simulink model "Thermal_Plant_model"  (R2025b)
settings: Solver=FixedStepDiscrete  StartTime=0.0  StopTime=200  FixedStep=0.1  RelTol=1e-3
libraries: slpidlib x4
settings Model: Creator=MFM  LastModifiedBy=MFM

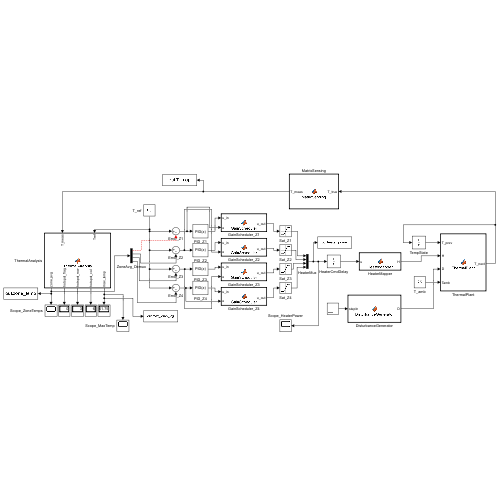
[thumbnail: Simulink's stored preview of the top-level diagram]
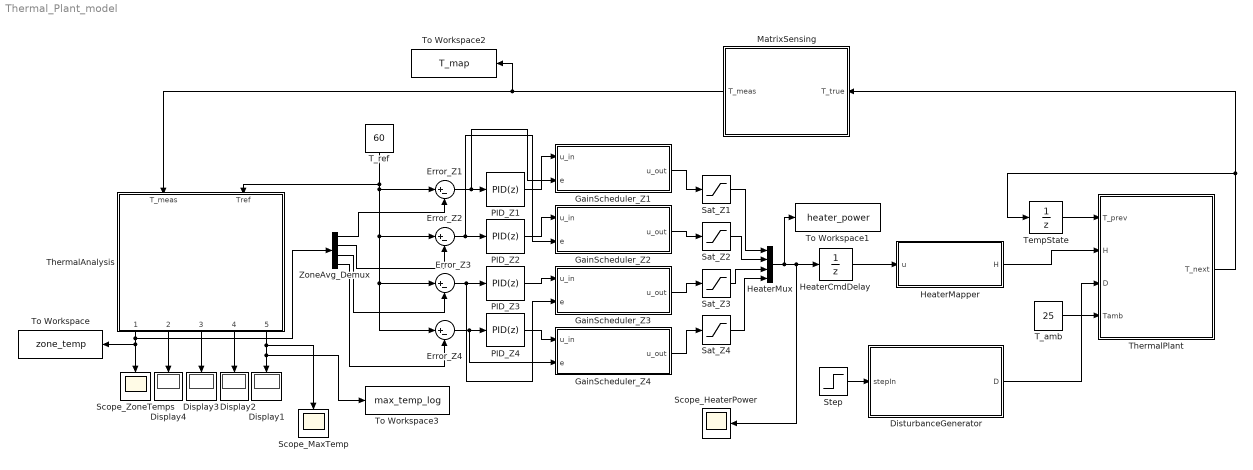
== system Thermal_Plant_model ==
  Display{1..4} (4 alike) : Display
  DisturbanceGenerator : MATLAB Function  TreatAsAtomicUnit=on
  Error_Z{1..4} (4 alike) : Sum  Inputs=|+-
  GainScheduler_Z1 : MATLAB Function  TreatAsAtomicUnit=on
  GainScheduler_Z2 : MATLAB Function  TreatAsAtomicUnit=on
  GainScheduler_Z3 : MATLAB Function  TreatAsAtomicUnit=on
  GainScheduler_Z4 : MATLAB Function  TreatAsAtomicUnit=on
  HeaterCmdDelay : UnitDelay  InitialCondition=[0 0 0 0]  SampleTime=-1  HasFrameUpgradeWarning=on
  HeaterMapper : MATLAB Function  TreatAsAtomicUnit=on
  HeaterMux : Mux
  MatrixSensing : MATLAB Function  TreatAsAtomicUnit=on
  PID_Z1 : slpidlib/PID Controller  Controller=PID  Form=Parallel  TimeDomain=Discrete-time  UseExternalTs=off  SampleTime=0.1  IntegratorMethod=Forward Euler  FilterMethod=Forward Euler  ControllerParametersSource=internal  P=2.5  I=1.2  UseKiTs=off  D=0.000  UseExternalDerivativeSource=off  N=100  UseFilter=on  TunerSelectOption=Transfer Function Based (PID Tuner App)  InitialConditionSource=internal  InitialConditionForIntegrator=0  InitialConditionForFilter=0  DifferentiatorICPrevScaledInput=0  ExternalReset=none  TrackingMode=off  Kt=1  LimitOutput=off  SatLimitsSource=internal  UpperSaturationLimit=inf  LowerSaturationLimit=-inf  LinearizeAsGain=on  AntiWindupMode=none  Kb=1  LimitIntegrator=off  UpperIntegratorSaturationLimit=inf  LowerIntegratorSaturationLimit=-inf  POutMin=[]  POutMax=[]  IOutMin=[]  IOutMax=[]  DOutMin=[]  DOutMax=[]  NOutMin=[]  NOutMax=[]  SumOutMin=[]  SumOutMax=[]  SaturationOutMin=[]  SaturationOutMax=[]  PParamMin=[]  PParamMax=[]  IParamMin=[]  IParamMax=[]  DParamMin=[]  DParamMax=[]  NParamMin=[]  NParamMax=[]  KbParamMin=[]  KbParamMax=[]  KtParamMin=[]  KtParamMax=[]  KbOutMin=[]  KbOutMax=[]  KtOutMin=[]  KtOutMax=[]  IntegratorOutMin=[]  IntegratorOutMax=[]  FilterOutMin=[]  FilterOutMax=[]  SumI1OutMin=[]  SumI1OutMax=[]  SumI2OutMin=[]  SumI2OutMax=[]  SumI3OutMin=[]  SumI3OutMax=[]  SumI4OutMin=[]  SumI4OutMax=[]  SumDOutMin=[]  SumDOutMax=[]  DifferentiatorOutMin=[]  DifferentiatorOutMax=[]  FilterDiffOutCoefMin=[]  FilterDiffOutCoefMax=[]  ReciprocalOutMin=[]  ReciprocalOutMax=[]  SumDenOutMin=[]  SumDenOutMax=[]  SumNumOutMin=[]  SumNumOutMax=[]  DivideOutMin=[]  DivideOutMax=[]  UdiffTsProdOutMin=[]  UdiffTsProdOutMax=[]  NTsProdOutMin=[]  NTsProdOutMax=[]  UintegralTsProdOutMin=[]  UintegralTsProdOutMax=[]  UngainTsProdOutMin=[]  UngainTsProdOutMax=[]  ClampingZeroOutDataTypeStr=Inherit: Inherit via back propagation  ClampingZeroOutMin=[]  ClampingZeroOutMax=[]  FilterDenConstantOutDataTypeStr=Inherit: Inherit via back propagation  FilterDenConstantOutMin=[]  FilterDenConstantOutMax=[]  PCopyOutDataTypeStr=Inherit: Inherit via back propagation  PCopyOutMin=[]  PCopyOutMax=[]  NCopyOutDataTypeStr=Inherit: Inherit via back propagation  NCopyOutMin=[]  NCopyOutMax=[]  IntegratorContinuousStateAttributes=''  IntegratorStateMustResolveToSignalObject=off  IntegratorRTWStateStorageClass=Auto  FilterContinuousStateAttributes=''  FilterStateMustResolveToSignalObject=off  FilterRTWStateStorageClass=Auto  ParallelPVariant=InternalParameters  IdealPVariant=Disabled  IVariant=InternalParameters  DVariant=InternalParameters  IntegratorVariant=Discrete  SatVariant=Disabled  AWVariant=Passthrough  PCopyVariant=Disabled  TRVariant=Disabled  FdbkBlocksVariant=Forward  IdealPFdbkVariant=Disabled  SatFdbkVariant=Disabled  DerivativeFilterVariant=ForwardEulerFilter  NVariant=InternalParameters  NCopyVariant=Disabled  FilterICVariant=InternalICsFilter  IntegratorICVariant=InternalICs  ExternalResetVariant=Disabled  TRSumVariant=Passthrough  SumFdbkVariant=Disabled  SumVariant=Sum_PID  TsampFilterVariant=InternalTs  TsampNgainVariant=Passthrough  TsampIntegralVariant=Disabled_SignalSpec  ExternalSaturationOutDataTypeStr=Inherit: Same as second input  DerivativeSourceVariant=ErrorSignal  PreIntVariant=InternalPreInt
  PID_Z2 : slpidlib/PID Controller  Controller=PID  Form=Parallel  TimeDomain=Discrete-time  UseExternalTs=off  SampleTime=0.1  IntegratorMethod=Forward Euler  FilterMethod=Forward Euler  ControllerParametersSource=internal  P=2.5  I=1.2  UseKiTs=off  D=0.0  UseExternalDerivativeSource=off  N=100  UseFilter=on  TunerSelectOption=Transfer Function Based (PID Tuner App)  InitialConditionSource=internal  InitialConditionForIntegrator=0  InitialConditionForFilter=0  DifferentiatorICPrevScaledInput=0  ExternalReset=none  TrackingMode=off  Kt=1  LimitOutput=off  SatLimitsSource=internal  UpperSaturationLimit=inf  LowerSaturationLimit=-inf  LinearizeAsGain=on  AntiWindupMode=none  Kb=1  LimitIntegrator=off  UpperIntegratorSaturationLimit=inf  LowerIntegratorSaturationLimit=-inf  POutMin=[]  POutMax=[]  IOutMin=[]  IOutMax=[]  DOutMin=[]  DOutMax=[]  NOutMin=[]  NOutMax=[]  SumOutMin=[]  SumOutMax=[]  SaturationOutMin=[]  SaturationOutMax=[]  PParamMin=[]  PParamMax=[]  IParamMin=[]  IParamMax=[]  DParamMin=[]  DParamMax=[]  NParamMin=[]  NParamMax=[]  KbParamMin=[]  KbParamMax=[]  KtParamMin=[]  KtParamMax=[]  KbOutMin=[]  KbOutMax=[]  KtOutMin=[]  KtOutMax=[]  IntegratorOutMin=[]  IntegratorOutMax=[]  FilterOutMin=[]  FilterOutMax=[]  SumI1OutMin=[]  SumI1OutMax=[]  SumI2OutMin=[]  SumI2OutMax=[]  SumI3OutMin=[]  SumI3OutMax=[]  SumI4OutMin=[]  SumI4OutMax=[]  SumDOutMin=[]  SumDOutMax=[]  DifferentiatorOutMin=[]  DifferentiatorOutMax=[]  FilterDiffOutCoefMin=[]  FilterDiffOutCoefMax=[]  ReciprocalOutMin=[]  ReciprocalOutMax=[]  SumDenOutMin=[]  SumDenOutMax=[]  SumNumOutMin=[]  SumNumOutMax=[]  DivideOutMin=[]  DivideOutMax=[]  UdiffTsProdOutMin=[]  UdiffTsProdOutMax=[]  NTsProdOutMin=[]  NTsProdOutMax=[]  UintegralTsProdOutMin=[]  UintegralTsProdOutMax=[]  UngainTsProdOutMin=[]  UngainTsProdOutMax=[]  ClampingZeroOutDataTypeStr=Inherit: Inherit via back propagation  ClampingZeroOutMin=[]  ClampingZeroOutMax=[]  FilterDenConstantOutDataTypeStr=Inherit: Inherit via back propagation  FilterDenConstantOutMin=[]  FilterDenConstantOutMax=[]  PCopyOutDataTypeStr=Inherit: Inherit via back propagation  PCopyOutMin=[]  PCopyOutMax=[]  NCopyOutDataTypeStr=Inherit: Inherit via back propagation  NCopyOutMin=[]  NCopyOutMax=[]  IntegratorContinuousStateAttributes=''  IntegratorStateMustResolveToSignalObject=off  IntegratorRTWStateStorageClass=Auto  FilterContinuousStateAttributes=''  FilterStateMustResolveToSignalObject=off  FilterRTWStateStorageClass=Auto  ParallelPVariant=InternalParameters  IdealPVariant=Disabled  IVariant=InternalParameters  DVariant=InternalParameters  IntegratorVariant=Discrete  SatVariant=Disabled  AWVariant=Passthrough  PCopyVariant=Disabled  TRVariant=Disabled  FdbkBlocksVariant=Forward  IdealPFdbkVariant=Disabled  SatFdbkVariant=Disabled  DerivativeFilterVariant=ForwardEulerFilter  NVariant=InternalParameters  NCopyVariant=Disabled  FilterICVariant=InternalICsFilter  IntegratorICVariant=InternalICs  ExternalResetVariant=Disabled  TRSumVariant=Passthrough  SumFdbkVariant=Disabled  SumVariant=Sum_PID  TsampFilterVariant=InternalTs  TsampNgainVariant=Passthrough  TsampIntegralVariant=Disabled_SignalSpec  ExternalSaturationOutDataTypeStr=Inherit: Same as second input  DerivativeSourceVariant=ErrorSignal  PreIntVariant=InternalPreInt
  PID_Z3 : slpidlib/PID Controller  Controller=PID  Form=Parallel  TimeDomain=Discrete-time  UseExternalTs=off  SampleTime=0.1  IntegratorMethod=Forward Euler  FilterMethod=Forward Euler  ControllerParametersSource=internal  P=2.5  I=1.2  UseKiTs=off  D=0  UseExternalDerivativeSource=off  N=100  UseFilter=on  TunerSelectOption=Transfer Function Based (PID Tuner App)  InitialConditionSource=internal  InitialConditionForIntegrator=0  InitialConditionForFilter=0  DifferentiatorICPrevScaledInput=0  ExternalReset=none  TrackingMode=off  Kt=1  LimitOutput=off  SatLimitsSource=internal  UpperSaturationLimit=inf  LowerSaturationLimit=-inf  LinearizeAsGain=on  AntiWindupMode=none  Kb=1  LimitIntegrator=off  UpperIntegratorSaturationLimit=inf  LowerIntegratorSaturationLimit=-inf  POutMin=[]  POutMax=[]  IOutMin=[]  IOutMax=[]  DOutMin=[]  DOutMax=[]  NOutMin=[]  NOutMax=[]  SumOutMin=[]  SumOutMax=[]  SaturationOutMin=[]  SaturationOutMax=[]  PParamMin=[]  PParamMax=[]  IParamMin=[]  IParamMax=[]  DParamMin=[]  DParamMax=[]  NParamMin=[]  NParamMax=[]  KbParamMin=[]  KbParamMax=[]  KtParamMin=[]  KtParamMax=[]  KbOutMin=[]  KbOutMax=[]  KtOutMin=[]  KtOutMax=[]  IntegratorOutMin=[]  IntegratorOutMax=[]  FilterOutMin=[]  FilterOutMax=[]  SumI1OutMin=[]  SumI1OutMax=[]  SumI2OutMin=[]  SumI2OutMax=[]  SumI3OutMin=[]  SumI3OutMax=[]  SumI4OutMin=[]  SumI4OutMax=[]  SumDOutMin=[]  SumDOutMax=[]  DifferentiatorOutMin=[]  DifferentiatorOutMax=[]  FilterDiffOutCoefMin=[]  FilterDiffOutCoefMax=[]  ReciprocalOutMin=[]  ReciprocalOutMax=[]  SumDenOutMin=[]  SumDenOutMax=[]  SumNumOutMin=[]  SumNumOutMax=[]  DivideOutMin=[]  DivideOutMax=[]  UdiffTsProdOutMin=[]  UdiffTsProdOutMax=[]  NTsProdOutMin=[]  NTsProdOutMax=[]  UintegralTsProdOutMin=[]  UintegralTsProdOutMax=[]  UngainTsProdOutMin=[]  UngainTsProdOutMax=[]  ClampingZeroOutDataTypeStr=Inherit: Inherit via back propagation  ClampingZeroOutMin=[]  ClampingZeroOutMax=[]  FilterDenConstantOutDataTypeStr=Inherit: Inherit via back propagation  FilterDenConstantOutMin=[]  FilterDenConstantOutMax=[]  PCopyOutDataTypeStr=Inherit: Inherit via back propagation  PCopyOutMin=[]  PCopyOutMax=[]  NCopyOutDataTypeStr=Inherit: Inherit via back propagation  NCopyOutMin=[]  NCopyOutMax=[]  IntegratorContinuousStateAttributes=''  IntegratorStateMustResolveToSignalObject=off  IntegratorRTWStateStorageClass=Auto  FilterContinuousStateAttributes=''  FilterStateMustResolveToSignalObject=off  FilterRTWStateStorageClass=Auto  ParallelPVariant=InternalParameters  IdealPVariant=Disabled  IVariant=InternalParameters  DVariant=InternalParameters  IntegratorVariant=Discrete  SatVariant=Disabled  AWVariant=Passthrough  PCopyVariant=Disabled  TRVariant=Disabled  FdbkBlocksVariant=Forward  IdealPFdbkVariant=Disabled  SatFdbkVariant=Disabled  DerivativeFilterVariant=ForwardEulerFilter  NVariant=InternalParameters  NCopyVariant=Disabled  FilterICVariant=InternalICsFilter  IntegratorICVariant=InternalICs  ExternalResetVariant=Disabled  TRSumVariant=Passthrough  SumFdbkVariant=Disabled  SumVariant=Sum_PID  TsampFilterVariant=InternalTs  TsampNgainVariant=Passthrough  TsampIntegralVariant=Disabled_SignalSpec  ExternalSaturationOutDataTypeStr=Inherit: Same as second input  DerivativeSourceVariant=ErrorSignal  PreIntVariant=InternalPreInt
  PID_Z4 : slpidlib/PID Controller  Controller=PID  Form=Parallel  TimeDomain=Discrete-time  UseExternalTs=off  SampleTime=0.1  IntegratorMethod=Forward Euler  FilterMethod=Forward Euler  ControllerParametersSource=internal  P=2.5  I=1.2  UseKiTs=off  D=0  UseExternalDerivativeSource=off  N=100  UseFilter=on  TunerSelectOption=Transfer Function Based (PID Tuner App)  InitialConditionSource=internal  InitialConditionForIntegrator=0  InitialConditionForFilter=0  DifferentiatorICPrevScaledInput=0  ExternalReset=none  TrackingMode=off  Kt=1  LimitOutput=off  SatLimitsSource=internal  UpperSaturationLimit=inf  LowerSaturationLimit=-inf  LinearizeAsGain=on  AntiWindupMode=none  Kb=1  LimitIntegrator=off  UpperIntegratorSaturationLimit=inf  LowerIntegratorSaturationLimit=-inf  POutMin=[]  POutMax=[]  IOutMin=[]  IOutMax=[]  DOutMin=[]  DOutMax=[]  NOutMin=[]  NOutMax=[]  SumOutMin=[]  SumOutMax=[]  SaturationOutMin=[]  SaturationOutMax=[]  PParamMin=[]  PParamMax=[]  IParamMin=[]  IParamMax=[]  DParamMin=[]  DParamMax=[]  NParamMin=[]  NParamMax=[]  KbParamMin=[]  KbParamMax=[]  KtParamMin=[]  KtParamMax=[]  KbOutMin=[]  KbOutMax=[]  KtOutMin=[]  KtOutMax=[]  IntegratorOutMin=[]  IntegratorOutMax=[]  FilterOutMin=[]  FilterOutMax=[]  SumI1OutMin=[]  SumI1OutMax=[]  SumI2OutMin=[]  SumI2OutMax=[]  SumI3OutMin=[]  SumI3OutMax=[]  SumI4OutMin=[]  SumI4OutMax=[]  SumDOutMin=[]  SumDOutMax=[]  DifferentiatorOutMin=[]  DifferentiatorOutMax=[]  FilterDiffOutCoefMin=[]  FilterDiffOutCoefMax=[]  ReciprocalOutMin=[]  ReciprocalOutMax=[]  SumDenOutMin=[]  SumDenOutMax=[]  SumNumOutMin=[]  SumNumOutMax=[]  DivideOutMin=[]  DivideOutMax=[]  UdiffTsProdOutMin=[]  UdiffTsProdOutMax=[]  NTsProdOutMin=[]  NTsProdOutMax=[]  UintegralTsProdOutMin=[]  UintegralTsProdOutMax=[]  UngainTsProdOutMin=[]  UngainTsProdOutMax=[]  ClampingZeroOutDataTypeStr=Inherit: Inherit via back propagation  ClampingZeroOutMin=[]  ClampingZeroOutMax=[]  FilterDenConstantOutDataTypeStr=Inherit: Inherit via back propagation  FilterDenConstantOutMin=[]  FilterDenConstantOutMax=[]  PCopyOutDataTypeStr=Inherit: Inherit via back propagation  PCopyOutMin=[]  PCopyOutMax=[]  NCopyOutDataTypeStr=Inherit: Inherit via back propagation  NCopyOutMin=[]  NCopyOutMax=[]  IntegratorContinuousStateAttributes=''  IntegratorStateMustResolveToSignalObject=off  IntegratorRTWStateStorageClass=Auto  FilterContinuousStateAttributes=''  FilterStateMustResolveToSignalObject=off  FilterRTWStateStorageClass=Auto  ParallelPVariant=InternalParameters  IdealPVariant=Disabled  IVariant=InternalParameters  DVariant=InternalParameters  IntegratorVariant=Discrete  SatVariant=Disabled  AWVariant=Passthrough  PCopyVariant=Disabled  TRVariant=Disabled  FdbkBlocksVariant=Forward  IdealPFdbkVariant=Disabled  SatFdbkVariant=Disabled  DerivativeFilterVariant=ForwardEulerFilter  NVariant=InternalParameters  NCopyVariant=Disabled  FilterICVariant=InternalICsFilter  IntegratorICVariant=InternalICs  ExternalResetVariant=Disabled  TRSumVariant=Passthrough  SumFdbkVariant=Disabled  SumVariant=Sum_PID  TsampFilterVariant=InternalTs  TsampNgainVariant=Passthrough  TsampIntegralVariant=Disabled_SignalSpec  ExternalSaturationOutDataTypeStr=Inherit: Same as second input  DerivativeSourceVariant=ErrorSignal  PreIntVariant=InternalPreInt
  Sat_Z{1..4} (4 alike) : Saturate  UpperLimit=100  LowerLimit=0
  Scope_HeaterPower : Scope
      settings: ActiveDisplayYMinimum=22.165592278395341  ActiveDisplayYMaximum=108.64826752462274
  Scope_MaxTemp : Scope
      settings: ActiveDisplayYMinimum=19.949054372354  ActiveDisplayYMaximum=70.261232158835853  DataLoggingVariableName=ScopeData2
  Scope_ZoneTemps : Scope
      settings: ActiveDisplayYMinimum=19.949054372354  ActiveDisplayYMaximum=70.261232158835853
  Step : Step  Time=10  SampleTime=0
  T_amb : Constant  Value=25
  T_ref : Constant  Value=60
  TempState : UnitDelay  InitialCondition=25*ones(6,8)  SampleTime=-1  HasFrameUpgradeWarning=on
  ThermalAnalysis : MATLAB Function  TreatAsAtomicUnit=on
  ThermalPlant : MATLAB Function  TreatAsAtomicUnit=on
  To Workspace : ToWorkspace  VariableName=zone_temp  SaveFormat=Structure With Time  SampleTime=-1
  To Workspace1 : ToWorkspace  VariableName=heater_power  SaveFormat=Structure With Time  SampleTime=-1
  To Workspace2 : ToWorkspace  VariableName=T_map  SaveFormat=Timeseries  SampleTime=-1
  To Workspace3 : ToWorkspace  VariableName=max_temp_log  SaveFormat=Structure With Time  SampleTime=-1
  ZoneAvg_Demux : Demux
  wires:
  T_ref/1 -> Error_Z3/1, Error_Z4/1, Error_Z2/1, Error_Z1/1, ThermalAnalysis/2(Tref)
  ZoneAvg_Demux/1 -> Error_Z1/2
  ZoneAvg_Demux/2 -> Error_Z2/2
  ZoneAvg_Demux/3 -> Error_Z3/2
  ZoneAvg_Demux/4 -> Error_Z4/2
  Sat_Z4/1 -> HeaterMux/4
  Sat_Z3/1 -> HeaterMux/3
  Sat_Z2/1 -> HeaterMux/2
  Sat_Z1/1 -> HeaterMux/1
  Step/1 -> DisturbanceGenerator/1(stepIn)
  T_amb/1 -> ThermalPlant/4(Tamb)
  TempState/1 -> ThermalPlant/1(T_prev)
  HeaterMapper/1(H) -> ThermalPlant/2(H)
  DisturbanceGenerator/1(D) -> ThermalPlant/3(D)
  ThermalPlant/1(T_next) -> TempState/1, MatrixSensing/1(T_true)
  MatrixSensing/1(T_meas) -> To Workspace2/1, ThermalAnalysis/1(T_meas)
  ThermalAnalysis/5(max_temp) -> Scope_MaxTemp/1, To Workspace3/1, Display1/1
  ThermalAnalysis/4(hotspot_col) -> Display2/1
  ThermalAnalysis/3(hotspot_row) -> Display3/1
  ThermalAnalysis/2(hotspot_flag) -> Display4/1
  Error_Z4/1 -> GainScheduler_Z4/2(e), PID_Z4/1
  Error_Z2/1 -> GainScheduler_Z2/2(e), PID_Z2/1
  Error_Z3/1 -> GainScheduler_Z3/2(e), PID_Z3/1
  Error_Z1/1 -> GainScheduler_Z1/2(e), PID_Z1/1
  HeaterMux/1 -> To Workspace1/1, Scope_HeaterPower/1, HeaterCmdDelay/1
  HeaterCmdDelay/1 -> HeaterMapper/1(u)
  ThermalAnalysis/1(zone_avg) -> Scope_ZoneTemps/1, To Workspace/1, ZoneAvg_Demux/1
  GainScheduler_Z1/1(u_out) -> Sat_Z1/1
  PID_Z1/1 -> GainScheduler_Z1/1(u_in)
  PID_Z2/1 -> GainScheduler_Z2/1(u_in)
  PID_Z3/1 -> GainScheduler_Z3/1(u_in)
  PID_Z4/1 -> GainScheduler_Z4/1(u_in)
  GainScheduler_Z2/1(u_out) -> Sat_Z2/1
  GainScheduler_Z3/1(u_out) -> Sat_Z3/1
  GainScheduler_Z4/1(u_out) -> Sat_Z4/1

== matlab function Thermal_Plant_model/ThermalAnalysis ==
  data: T_meas input; zone_avg output; Tref input; hotspot_flag output; hotspot_row output; hotspot_col output; max_temp output
function [zone_avg, hotspot_flag, hotspot_row, hotspot_col, max_temp] = ThermalAnalysis(T_meas,Tref)

zone_avg = zeros(1,4);

% Zone 1
zone_avg(1) = mean(mean(T_meas(1:3,1:4)));

% Zone 2
zone_avg(2) = mean(mean(T_meas(1:3,5:8)));

% Zone 3
zone_avg(3) = mean(mean(T_meas(4:6,1:4)));

% Zone 4
zone_avg(4) = mean(mean(T_meas(4:6,5:8)));

% Find maximum temperature
[max_temp, idx] = max(T_meas(:));
[hotspot_row, hotspot_col] = ind2sub(size(T_meas), idx);

% Hotspot definition
if max_temp > (Tref + 8)
    hotspot_flag = 1;
else
    hotspot_flag = 0;
end
end

== matlab function Thermal_Plant_model/ThermalPlant ==
  data: T_prev input; T_next output; H input; D input; Tamb input
function T_next = ThermalPlant(T_prev,H,D,Tamb)
% 6x8 thermal grid update
% T_prev : previous temperature matrix
% H      : heater input matrix
% D      : disturbance matrix
% Tamb   : ambient temperature

T_next = T_prev;

dt = 0.1;     % simulation time step
a = 0.15;     % lateral heat diffusion coefficient
b = 0.03;     % heater gain
c = 0.08;     % ambient heat loss coefficient
d = 0.05;     % disturbance gain

[rows, cols] = size(T_prev);

for i = 1:rows
    for j = 1:cols
        
        T_here = T_prev(i,j);
        neigh_sum = 0;
        neigh_count = 0;
        
        % Up
        if i > 1
            neigh_sum = neigh_sum + T_prev(i-1,j);
            neigh_count = neigh_count + 1;
        end
        
        % Down
        if i < rows
            neigh_sum = neigh_sum + T_prev(i+1,j);
            neigh_count = neigh_count + 1;
        end
        
        % Left
        if j > 1
            neigh_sum = neigh_sum + T_prev(i,j-1);
            neigh_count = neigh_count + 1;
        end
        
        % Right
        if j < cols
            neigh_sum = neigh_sum + T_prev(i,j+1);
            neigh_count = neigh_count + 1;
        end
        
        diffusion = a * (neigh_sum - neigh_count*T_here);
        heater = b * H(i,j);
        disturb = d * D(i,j);
        ambient_loss = -c * (T_here - Tamb);
        
        dT = diffusion + heater + disturb + ambient_loss;
        
        T_next(i,j) = T_here + dt*dT;
    end
end
end

== matlab function Thermal_Plant_model/DisturbanceGenerator ==
  data: stepIn input; D output
function D = DisturbanceGenerator(stepIn)
% Disturbance matrix, activated after stepIn becomes 1

D = zeros(6,8);

if stepIn > 0.5
    % Example hotspot disturbance in upper-right area
    D(2:3,6:7) = 20;
end
end

== matlab function Thermal_Plant_model/MatrixSensing ==
  data: T_true input; T_meas output
function T_meas = MatrixSensing(T_true)
% Simulated matrix-based sensing
% For simplicity, return same matrix with tiny measurement noise

noise_amp = 0.05;  % small noise
T_meas = T_true + noise_amp*randn(6,8);
end

== matlab function Thermal_Plant_model/HeaterMapper ==
  data: u input; H output
function H = HeaterMapper(u)
% u = [u1 u2 u3 u4]% Output H is a 6x8 heater matrix

H = zeros(6,8);

% Zone 1: rows 1:3, cols 1:4
H(1:3,1:4) = u(1);

% Zone 2: rows 1:3, cols 5:8
H(1:3,5:8) = u(2);

% Zone 3: rows 4:6, cols 1:4
H(4:6,1:4) = u(3);

% Zone 4: rows 4:6, cols 5:8
H(4:6,5:8) = u(4);
end

== matlab function Thermal_Plant_model/GainScheduler_Z1 ==
  data: u_in input; u_out output; e input
function u_out = GainScheduler(u_in, e)
% Error-dependent output scaling

ae = abs(e);

if ae > 8
    g = 0.9;     % aggressive heating when far from setpoint
elseif ae > 2
    g = 1.1;     % normal control
else
    g = 0.5;     % softer action near setpoint
end

u_out = g * u_in;
end

== matlab function Thermal_Plant_model/GainScheduler_Z2 ==
  data: u_in input; u_out output; e input
function u_out = GainScheduler(u_in, e)
% Error-dependent output scaling

ae = abs(e);

if ae > 8
    g = 0.9;     % aggressive heating when far from setpoint
elseif ae > 2
    g = 1.1;     % normal control
else
    g = 0.5;     % softer action near setpoint
end

u_out = g * u_in;
end

== matlab function Thermal_Plant_model/GainScheduler_Z3 ==
  data: u_in input; u_out output; e input
function u_out = GainScheduler(u_in, e)
% Error-dependent output scaling

ae = abs(e);

if ae > 8
    g = 0.9;     % aggressive heating when far from setpoint
elseif ae > 2
    g = 1.1;     % normal control
else
    g = 0.5;     % softer action near setpoint
end

u_out = g * u_in;
end

== matlab function Thermal_Plant_model/GainScheduler_Z4 ==
  data: u_in input; u_out output; e input
function u_out = GainScheduler(u_in, e)
% Error-dependent output scaling

ae = abs(e);

if ae > 8
    g = 0.9;     % aggressive heating when far from setpoint
elseif ae > 2
    g = 1.1;     % normal control
else
    g = 0.5;     % softer action near setpoint
end

u_out = g * u_in;
end
